simulink model "untitled"  (R2026a)
settings: Solver=VariableStepAuto
libraries: dspfdesign x1
settings Model: Creator=GIGABYTE  LastModifiedBy=GIGABYTE

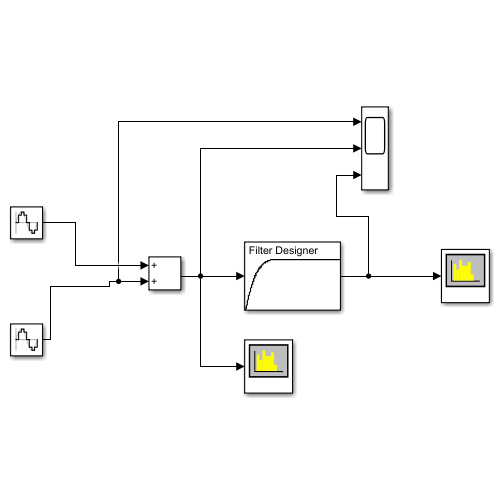
[thumbnail: Simulink's stored preview of the top-level diagram]
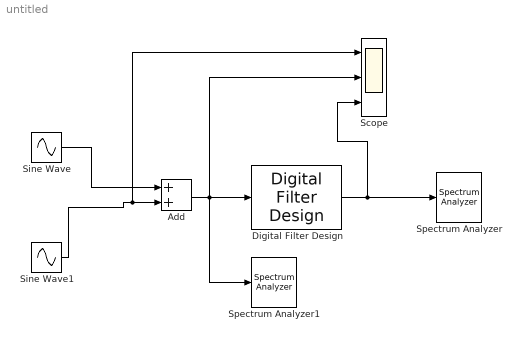
== system untitled ==
  Add : Sum
  Digital Filter Design : dspfdesign/Digital Filter Design  mwdsp_browser_bugfix_var=off
  Scope : Scope  NumInputPorts=3
      settings: ActiveDisplayYMinimum=-1.2500000000000009  ActiveDisplayYMaximum=1.2500000000000007
  Sine Wave : Sin  Frequency=1000*2*pi  SampleTime=1/100000
  Sine Wave1 : Sin  Frequency=10000*2*pi  SampleTime=1/100000
  Spectrum Analyzer : SpectrumAnalyzer  WindowPosition=[1.000000,49.000000,1536.000000,889.000000,]  ScopeFrameLocation=window  WindowInvariantSamplesPerUpdate=on  YLimits=[-357.98420000000004 254.55260000000004]
  Spectrum Analyzer1 : SpectrumAnalyzer  WindowPosition=[368.000000,230.000000,800.000000,500.000000,]  ScopeFrameLocation=window  WindowInvariantSamplesPerUpdate=on  YLimits=[-248.9518 54.2754]
  wires:
  Sine Wave/1 -> Add/1
  Sine Wave1/1 -> Scope/1, Add/2
  Add/1 -> Scope/2, Digital Filter Design/1, Spectrum Analyzer1/1
  Digital Filter Design/1 -> Scope/3, Spectrum Analyzer/1
